simulink model "furuta"  (R2021a)
settings: Solver=ode45  StartTime=0.0  StopTime=5  MaxStep=0.001  RelTol=1e-9  AbsTol=1e-9
values from neighbouring files (symbols this model uses):
  A_up = double([0,0,1,0 ... (first row only)    [cw_furuta.m]    (also in lin_systems.mat = [0 0 0 0 0 0 52.8369133028 98.0815161146 1 0 -19.5069283319 ; matrices.mat = [0 0 0 0 0 0 52.8369133028 98.0815161146 1 0 -19.5069283319 )
  B_up = double([0 ... (first row only)    [cw_furuta.m]    (also in lin_systems.mat = [0 0 35.0660473259 34.9971460369]; matrices.mat = [0 0 35.0660473259 34.9971460369])
  K_lqr_u = [-0.01 12.6268987044 -1.12531130243 1.5627946446]    [matrices.mat]
  x0 = [pi-0.1 ... (first row only)    [cw_furuta.m]    (also in matrices.mat = [3.04159265359 0.392699081699 0.3 0.1])
settings Model: Creator=filippo  LastModifiedBy=filippo

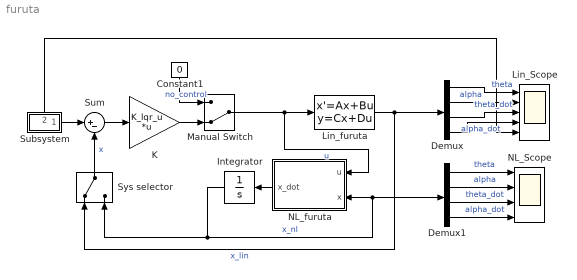
== system furuta ==
  Constant1 : Constant  Value=0
  Demux : Demux
  Demux1 : Demux
  Integrator : Integrator  InitialCondition=x0
  K : Gain  Gain=K_lqr_u  Multiplication=Matrix(K*u) (u vector)
  Lin_Scope : Scope  NumInputPorts=5
  Lin_furuta : StateSpace  A=A_up  B=B_up  C=eye(4)  D=zeros(4,1)  InitialCondition=x0
  Manual Switch : ManualSwitch  CurrentSetting=0
  NL_Scope : Scope  NumInputPorts=4
  NL_furuta : MATLAB Function  TreatAsAtomicUnit=on
  Subsystem : Subsystem
      settings: PortSchema="{\"entries\":[{\"content\":{\"sides\":[{\"content\":{\"connectorIds\":[]},\"type\":\"ConnectorPlacement.EquallySpacedRectSide\",\"uuid\":\"c057468e-68cb-4a4b-9ead-048d1f61513c\"},{\"content\":{\"connectorIds\":[\"Out1\"],\"side\":\"RIGHT\"},\"type\":\"ConnectorPlacement.EquallySpacedRectSide\",\"uuid\":\"4c06bb7f-fdee-4161-ab60-9c40ed3a53b2\"},{\"content\":{\"connectorIds\":[\"Out2\"],\"side\":\"TOP\"},\"type\":\"ConnectorPlacement.EquallySpacedRectSide\",\"uuid\":\"462cfa0f-89b3-4415-9d46-c05857bcb7b8\"}]},\"type\":\"ConnectorPlacement.EquallySpacedConnector\",\"uuid\":\"637880ca-3b27-4e8a-bf6b-b2519e94e1cc\"}],\"packageUris\":[\"http://schema.mathworks.com/mf0/Connector/R2020b\"],\"version\":\"1.0\"}"
  Sum : Sum  Inputs=|+-
  Sys selector : ManualSwitch
  wires:
  Lin_furuta/1 -> Demux/1, Sys selector/1  "x_lin"
  Sum/1 -> K/1
  K/1 -> Manual Switch/2
  Demux/1 -> Lin_Scope/1  "theta"
  Demux/2 -> Lin_Scope/2  "alpha"
  Demux/3 -> Lin_Scope/3  "theta_dot"
  Demux/4 -> Lin_Scope/4  "alpha_dot"
  Constant1/1 -> Manual Switch/1  "no_control"
  Manual Switch/1 -> Lin_furuta/1, NL_furuta/1(u)  "u"
  NL_furuta/1(x_dot) -> Integrator/1
  Demux1/2 -> NL_Scope/2  "alpha"
  Demux1/1 -> NL_Scope/1  "theta"
  Demux1/3 -> NL_Scope/3  "theta_dot"
  Integrator/1 -> Demux1/1, NL_furuta/2(x), Sys selector/2  "x_nl"
  Demux1/4 -> NL_Scope/4  "alpha_dot"
  Sys selector/1 -> Sum/2  "x"
  Subsystem/1(x_des) -> Sum/1
  Subsystem/2(alpha_ref) -> Lin_Scope/5

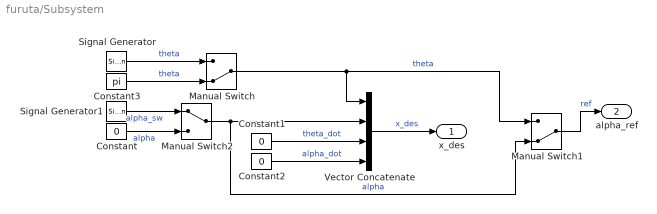
== system furuta/Subsystem ==
  Constant : Constant  Value=0
  Constant1 : Constant  Value=0
  Constant2 : Constant  Value=0
  Constant3 : Constant  Value=pi
  Manual Switch : ManualSwitch  CurrentSetting=0
  Manual Switch1 : ManualSwitch  CurrentSetting=0
  Manual Switch2 : ManualSwitch
  Signal Generator : SignalGenerator  WaveForm=square  Amplitude=deg2rad(45)  Frequency=(2*pi)  Units=rad/sec
  Signal Generator1 : SignalGenerator  WaveForm=square  Amplitude=deg2rad(45)  Frequency=10*(2*pi)  Units=rad/sec
  Vector Concatenate : Concatenate  NumInputs=4
  x_des : Outport
  alpha_ref : Outport  Port=2
  wires:
  Vector Concatenate/1 -> x_des/1  "x_des"
  Manual Switch2/1 -> Manual Switch1/2, Vector Concatenate/2  "alpha"
  Constant1/1 -> Vector Concatenate/3  "theta_dot"
  Constant2/1 -> Vector Concatenate/4  "alpha_dot"
  Constant3/1 -> Manual Switch/2  "theta"
  Signal Generator/1 -> Manual Switch/1  "theta"
  Manual Switch/1 -> Manual Switch1/1, Vector Concatenate/1  "theta"
  Signal Generator1/1 -> Manual Switch2/1  "alpha_sw"
  Constant/1 -> Manual Switch2/2  "alpha"
  Manual Switch1/1 -> alpha_ref/1  "ref"

== matlab function furuta/NL_furuta ==
  data: u input; x input; x_dot output
function x_dot = furuta(u,x)
% Furuta pendulum 

% renaming state in compliance with altready written code

% th = x(1); % not used variable, saving calculations
a = x(2); % x(2)+pi FOR UPWARD POSITION
th_d = x(3);
a_d = x(4);

% assigning values to symbolic values 

Rm = 2.6; Kt = 7.68e-3; Em = 0.69; Km = 7.68e-3; Kg = 70;
Eg = 0.9; mp = 0.127; lp = 0.1556; Jp = 0.0012; Jarm = 0.002;
Bp = 0.0024; Barm = 0.0024; r = 0.2159; g = 9.81;

% defining matrices

D = [(r^2)*mp+(lp^2)*mp-(lp^2)*(cos(a)^2)*mp+Jarm, r*cos(a)*mp*lp ;
    r*cos(a)*mp*lp                              , (lp^2)*mp+Jp      ];

C = [2*mp*cos(a)*a_d*(lp^2)*sin(a), -mp*sin(a)*a_d*lp*r;
    -mp*cos(a)*th_d*(lp^2)*sin(a) ,           0        ];

G = [     0; 
    mp*g*sin(a)*lp];

tau_m = Eg*Kg*Em*Kt*(u-Kg*Km*th_d)/Rm;

tau = [tau_m - Barm*th_d;
            -Bp*a_d     ];

% defining the non-linear equations
x_dot  = zeros(4,1);

x_dot(1:2) = [th_d;
               a_d]; 

x_dot(3:4) = (D^-1)*(tau - G - C*[th_d; a_d]);

end
